simulink model "right_shoulder_sine"  (Simulink 7.7)
settings: Solver=FixedStepDiscrete  StartTime=0.0  StopTime=20.0  FixedStep=0.05  RelTol=1e-3
undefined symbols (not defined in the file): darwinop_communication_setup
libraries: lib_darwinop x3
settings Model: Creator=florent  LastModifiedBy=eleve
settings DataIOCC: SignalLoggingSaveFormat=Dataset
settings OptimizationCC: ExpressionDepthLimit=128  OptimizeModelRefInitCode=on  LifeSpan=1
settings DebuggingCC: FcnCallInpInsideContextMsg=Enable All
settings HardwareCC: ProdEndianess=LittleEndian  ProdHWDeviceType=Generic->32-bit Embedded Processor
settings RTWCC: SystemTargetFile=darwinoplib.tlc  GenCodeOnly=on  TemplateMakefile=darwinoplib.tmf  Description=DarwinOP code generator  ProcessScript=darwinoplib_make_rtw_hook  TargetLang=C++
settings CodeAppCC: IgnoreCustomStorageClasses=off  CustomSymbolStrType=$N$R$M_T
settings STFCustomTargetCC: CombineOutputUpdateFcns=on  ERTCustomFileBanners=on  SupportContinuousTime=off  SupportNonInlinedSFcns=off  SystemTargetFile=darwinoplib.tlc
settings ERTTargetCC: MultiwordLength=2048  ParMdlRefBuildCompliant=off  CompOptLevelCompliant=off  ERTFirstTimeCompliant=off  ModelStepFunctionPrototypeControlCompliant=off  CPPClassGenCompliant=off  ExtModeMexArgs='192.168.123.1' 1 17725  InlinedParameterPlacement=NonHierarchical  ERTCustomFileTemplate=darwinoplib_main.tlc  ConvertIfToSwitch=off  SuppressUnreachableDefaultCases=off
settings CustomProperty: DataType=string  Value=192.168.123.1

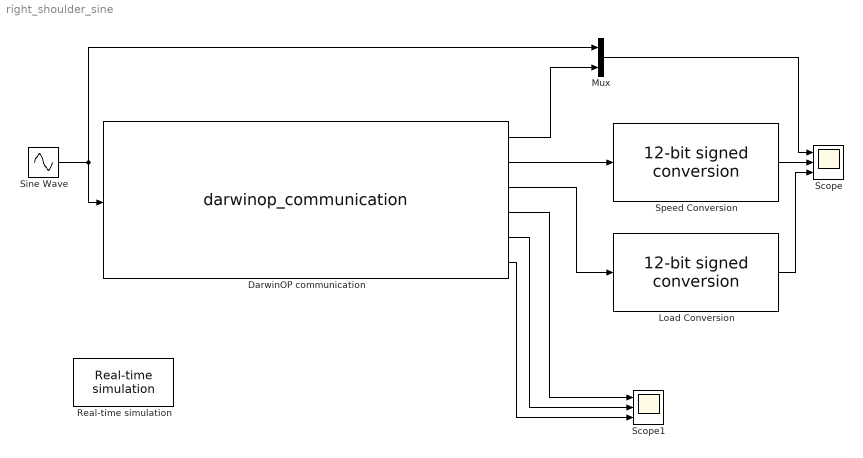
== system right_shoulder_sine ==
  DarwinOP communication : M-S-Function  StartFcn=darwinop_communication_setup('StartFcn');  StopFcn=darwinop_communication_setup('StopFcn');  FunctionName=darwinop_communication  Parameters=IP,Port,Protocol,Timeout,Frame,ReadIndex,WriteIndex  mask{IP=192.168.123.1, Port=1234, Protocol=tcp, Timeout=0.05, Frame=[ 2 1 36 6 3 1 30 2 0 0 2 200 44 6], ReadIndex=[ 1 2;3 2;5 2;7 2;9 2;11 2], WriteIndex=[ 9 2]}
      settings: DeleteFcn=darwinop_communication_setup('DeleteFcn');  ModelCloseFcn=darwinop_communication_setup('ModelCloseFcn');  NameChangeFcn=darwinop_communication_setup('NameChangeFcn');  OpenFcn=darwinop_communication_setup('OpenFcn');
      mask StyleString: edit,edit,popup(tcp|udp),edit,edit,edit,edit
      mask Display:
      | image(imread('darwin-blk.jpg'))
      | 
      | port_label('output',1,'Right Shoulder Pitch(1)/Position')
      | port_label('output',2,'Right Shoulder Pitch(1)/Speed')
      | port_label('output',3,'Right Shoulder Pitch(1)/Load')
      | port_label('output',4,'Sub controller(200)/ACC X')
      | port_label('output',5,'Sub controller(200)/ACC Y')
      | port_label('output',6,'Sub controller(200)/ACC Z')
      | 
      | port_label('input',1,'Right Shoulder Pitch(1)/Goal Position')
  Load Conversion : lib_darwinop/12-bit signed conversion
  Mux : Mux  Inputs=2
  Real-time simulation : lib_darwinop/Real-time simulation  TimeScalingFactor=1
  Scope : Scope  NumInputPorts=3
      settings: YMin=1000~-100~-700  YMax=3000~475~200
  Scope1 : Scope  NumInputPorts=3
      settings: YMin=507~505~622.5  YMax=519~535~655
  Sine Wave : Sin  Amplitude=1000  Bias=2000  SampleTime=0.05
  Speed Conversion : lib_darwinop/12-bit signed conversion
  wires:
  Sine Wave/1 -> DarwinOP communication/1, Mux/1
  DarwinOP communication/1 -> Mux/2
  DarwinOP communication/3 -> Load Conversion/1
  DarwinOP communication/2 -> Speed Conversion/1
  Speed Conversion/1 -> Scope/2
  Load Conversion/1 -> Scope/3
  Mux/1 -> Scope/1
  DarwinOP communication/4 -> Scope1/1
  DarwinOP communication/5 -> Scope1/2
  DarwinOP communication/6 -> Scope1/3
